simulink model "DC_motor"  (R2019a)
settings: Solver=VariableStepAuto  StartTime=0.0  StopTime=10.0  RelTol=1e-3
values from neighbouring files (symbols this model uses):
  b = 0.1    [DC_Motor.m]
  J = 0.01    [DC_Motor.m]
  K = 0.01    [DC_Motor.m]
  L = 0.5    [DC_Motor.m]
  R = 1    [DC_Motor.m]
settings Model: Creator=ragha  LastModifiedBy=ragha

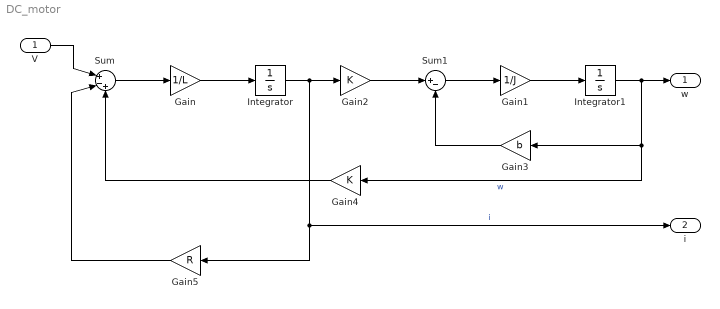
== system DC_motor ==
  V : Inport
  Gain : Gain  Gain=1/L
  Gain1 : Gain  Gain=1/J
  Gain2 : Gain  Gain=K
  Gain3 : Gain  Gain=b
  Gain4 : Gain  Gain=K
  Gain5 : Gain  Gain=R
  Integrator : Integrator
  Integrator1 : Integrator
  Sum : Sum  Inputs=|+-+
  Sum1 : Sum  Inputs=|+-
  w : Outport
  i : Outport  Port=2
  wires:
  Sum1/1 -> Gain1/1
  Gain1/1 -> Integrator1/1
  Integrator/1 -> Gain5/1, i/1, Gain2/1  "i"
  Gain2/1 -> Sum1/1
  Gain3/1 -> Sum1/2
  Integrator1/1 -> Gain4/1, Gain3/1, w/1  "w"
  Gain4/1 -> Sum/3
  Gain5/1 -> Sum/2
  Sum/1 -> Gain/1
  Gain/1 -> Integrator/1
  V/1 -> Sum/1
